simulink model "sistema"  (R2023a)
settings: Solver=ode23t  StartTime=0.0  StopTime=10.0  MaxStep=1e-3  RelTol=1e-6
libraries: fl_lib x18, nesl_utility x9, ee_lib x3, slpidlib x2
settings Model: Creator=Bricia Arellano  LastModifiedBy=Bricia Arellano
settings DataIOCC: ReturnWorkspaceOutputs=off  TimeSaveName=t
settings DebuggingCC: AlgebraicLoopMsg=none  ArtificialAlgebraicLoopMsg=none  MaxConsecutiveZCsMsg=none  ModelReferenceExtraNoncontSigs=none  OperatingPointInterfaceChecksumMismatchMsg=none

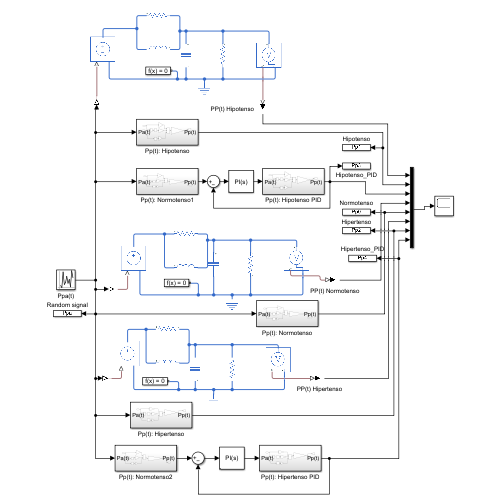
[thumbnail: Simulink's stored preview of the top-level diagram]
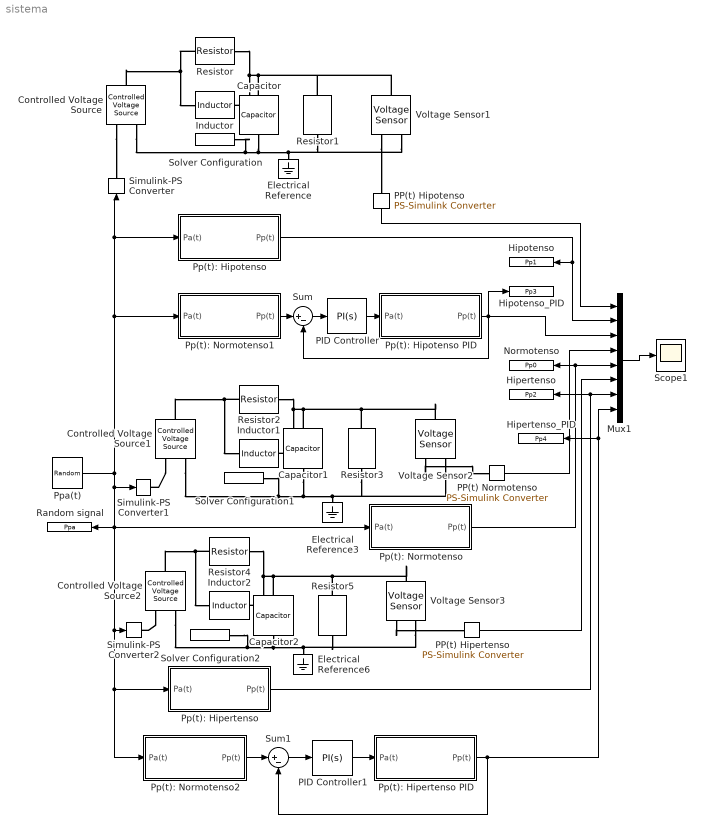
== system sistema ==
  Capacitor : fl_lib/Electrical/Electrical Elements/Capacitor  c=0.25 F  r=1e-6 Ohm  g=0 1/Ohm  i_specify=off  i_priority=None  i=0 A  i_nominal_specify=off  i_nominal_unit=A  i_nominal_value=1  v_specify=off  v_priority=None  v=0 V  v_nominal_specify=off  v_nominal_unit=V  v_nominal_value=1  vc_specify=off  vc_priority=High  vc=0 V  vc_nominal_specify=off  vc_nominal_unit=V  vc_nominal_value=1
  Capacitor1 : fl_lib/Electrical/Electrical Elements/Capacitor  c=1.5 F  r=1e-6 Ohm  g=0 1/Ohm  i_specify=off  i_priority=None  i=0 A  i_nominal_specify=off  i_nominal_unit=A  i_nominal_value=1  v_specify=off  v_priority=None  v=0 V  v_nominal_specify=off  v_nominal_unit=V  v_nominal_value=1  vc_specify=off  vc_priority=High  vc=0 V  vc_nominal_specify=off  vc_nominal_unit=V  vc_nominal_value=1
  Capacitor2 : fl_lib/Electrical/Electrical Elements/Capacitor  c=2.5 F  r=1e-6 Ohm  g=0 1/Ohm  i_specify=off  i_priority=None  i=0 A  i_nominal_specify=off  i_nominal_unit=A  i_nominal_value=1  v_specify=off  v_priority=None  v=0 V  v_nominal_specify=off  v_nominal_unit=V  v_nominal_value=1  vc_specify=off  vc_priority=High  vc=0 V  vc_nominal_specify=off  vc_nominal_unit=V  vc_nominal_value=1
  Controlled Voltage Source : fl_lib/Electrical/Electrical Sources/Controlled Voltage Source
  Controlled Voltage Source1 : fl_lib/Electrical/Electrical Sources/Controlled Voltage Source
  Controlled Voltage Source2 : fl_lib/Electrical/Electrical Sources/Controlled Voltage Source
  Electrical Reference : fl_lib/Electrical/Electrical Elements/Electrical Reference
  Electrical Reference3 : fl_lib/Electrical/Electrical Elements/Electrical Reference
  Electrical Reference6 : fl_lib/Electrical/Electrical Elements/Electrical Reference
  Hipertenso : ToWorkspace  VariableName=Pp2  SampleTime=-1
  Hipertenso_PID : ToWorkspace  VariableName=Pp4  SampleTime=-1
  Hipotenso : ToWorkspace  VariableName=Pp1  SampleTime=-1
  Hipotenso_PID : ToWorkspace  VariableName=Pp3  SampleTime=-1
  Inductor : ee_lib/Passive/Inductor  l=0.005 H  enable_L_tol=ee.enum.toleranceApplication.none  L_tol=20  tol_distribution=ee.enum.toleranceDistribution.uniform  nSigma=4  r=0 Ohm  g=1e-9 1/Ohm  enable_operating_limits=ee.enum.enable.no  operating_limit_action=ee.enum.passive.reportOpLim.warn  max_working_current=1 A  power_rating=1 W  enable_faults=ee.enum.enable.no  fault_action=simscape.enum.assert.action.none  lambdaPercent=50  k_faulted=0.9999  turnsShort=ee.enum.passive.inductor.turnsShortOption.no  openCct=ee.enum.enable.no  groundShort=ee.enum.passive.inductor.groundShortOption.no  groundShortG=0 1/Ohm  tau_fault=1e-3 s  fault_trigger=ee.enum.faults.faultTrigger.temporal  t_fault=1 s  max_permissible_voltage=100 V  n_fail_on_voltage=1  max_permissible_current=1 A  t_fail_on_current=1 s  i_L_specify=off  i_L_priority=High  i_L=0 A  i_L_nominal_specify=off  i_L_nominal_unit=A  i_L_nominal_value=1
  Inductor1 : ee_lib/Passive/Inductor  l=0.01 H  enable_L_tol=ee.enum.toleranceApplication.none  L_tol=20  tol_distribution=ee.enum.toleranceDistribution.uniform  nSigma=4  r=0 Ohm  g=1e-9 1/Ohm  enable_operating_limits=ee.enum.enable.no  operating_limit_action=ee.enum.passive.reportOpLim.warn  max_working_current=1 A  power_rating=1 W  enable_faults=ee.enum.enable.no  fault_action=simscape.enum.assert.action.none  lambdaPercent=50  k_faulted=0.9999  turnsShort=ee.enum.passive.inductor.turnsShortOption.no  openCct=ee.enum.enable.no  groundShort=ee.enum.passive.inductor.groundShortOption.no  groundShortG=0 1/Ohm  tau_fault=1e-3 s  fault_trigger=ee.enum.faults.faultTrigger.temporal  t_fault=1 s  max_permissible_voltage=100 V  n_fail_on_voltage=1  max_permissible_current=1 A  t_fail_on_current=1 s  i_L_specify=off  i_L_priority=High  i_L=0 A  i_L_nominal_specify=off  i_L_nominal_unit=A  i_L_nominal_value=1
  Inductor2 : ee_lib/Passive/Inductor  l=0.02 H  enable_L_tol=ee.enum.toleranceApplication.none  L_tol=20  tol_distribution=ee.enum.toleranceDistribution.uniform  nSigma=4  r=0 Ohm  g=1e-9 1/Ohm  enable_operating_limits=ee.enum.enable.no  operating_limit_action=ee.enum.passive.reportOpLim.warn  max_working_current=1 A  power_rating=1 W  enable_faults=ee.enum.enable.no  fault_action=simscape.enum.assert.action.none  lambdaPercent=50  k_faulted=0.9999  turnsShort=ee.enum.passive.inductor.turnsShortOption.no  openCct=ee.enum.enable.no  groundShort=ee.enum.passive.inductor.groundShortOption.no  groundShortG=0 1/Ohm  tau_fault=1e-3 s  fault_trigger=ee.enum.faults.faultTrigger.temporal  t_fault=1 s  max_permissible_voltage=100 V  n_fail_on_voltage=1  max_permissible_current=1 A  t_fail_on_current=1 s  i_L_specify=off  i_L_priority=High  i_L=0 A  i_L_nominal_specify=off  i_L_nominal_unit=A  i_L_nominal_value=1
  Mux1 : Mux  Inputs=8
  Normotenso : ToWorkspace  VariableName=Pp0  SampleTime=-1
  PID Controller : slpidlib/PID Controller  Controller=PI  Form=Parallel  TimeDomain=Continuous-time  UseExternalTs=off  SampleTime=-1  IntegratorMethod=Forward Euler  FilterMethod=Forward Euler  ControllerParametersSource=internal  P=4.21636346738391e-05  I=3267.68674685278  UseKiTs=off  D=0  N=100  UseFilter=on  TunerSelectOption=Transfer Function Based (PID Tuner App)  InitialConditionSource=internal  InitialConditionForIntegrator=0  InitialConditionForFilter=0  DifferentiatorICPrevScaledInput=0  ExternalReset=none  TrackingMode=off  Kt=1  LimitOutput=off  SatLimitsSource=internal  UpperSaturationLimit=inf  LowerSaturationLimit=-inf  LinearizeAsGain=on  AntiWindupMode=none  Kb=1  LimitIntegrator=off  UpperIntegratorSaturationLimit=inf  LowerIntegratorSaturationLimit=-inf  POutMin=[]  POutMax=[]  IOutMin=[]  IOutMax=[]  DOutMin=[]  DOutMax=[]  NOutMin=[]  NOutMax=[]  SumOutMin=[]  SumOutMax=[]  SaturationOutMin=[]  SaturationOutMax=[]  PParamMin=[]  PParamMax=[]  IParamMin=[]  IParamMax=[]  DParamMin=[]  DParamMax=[]  NParamMin=[]  NParamMax=[]  KbParamMin=[]  KbParamMax=[]  KtParamMin=[]  KtParamMax=[]  KbOutMin=[]  KbOutMax=[]  KtOutMin=[]  KtOutMax=[]  IntegratorOutMin=[]  IntegratorOutMax=[]  FilterOutMin=[]  FilterOutMax=[]  SumI1OutMin=[]  SumI1OutMax=[]  SumI2OutMin=[]  SumI2OutMax=[]  SumI3OutMin=[]  SumI3OutMax=[]  SumI4OutMin=[]  SumI4OutMax=[]  SumDOutMin=[]  SumDOutMax=[]  DifferentiatorOutMin=[]  DifferentiatorOutMax=[]  FilterDiffOutCoefMin=[]  FilterDiffOutCoefMax=[]  ReciprocalOutMin=[]  ReciprocalOutMax=[]  SumDenOutMin=[]  SumDenOutMax=[]  SumNumOutMin=[]  SumNumOutMax=[]  DivideOutMin=[]  DivideOutMax=[]  UdiffTsProdOutMin=[]  UdiffTsProdOutMax=[]  NTsProdOutMin=[]  NTsProdOutMax=[]  UintegralTsProdOutMin=[]  UintegralTsProdOutMax=[]  UngainTsProdOutMin=[]  UngainTsProdOutMax=[]  ClampingZeroOutDataTypeStr=Inherit: Inherit via back propagation  ClampingZeroOutMin=[]  ClampingZeroOutMax=[]  FilterDenConstantOutDataTypeStr=Inherit: Inherit via back propagation  FilterDenConstantOutMin=[]  FilterDenConstantOutMax=[]  PCopyOutDataTypeStr=Inherit: Inherit via back propagation  PCopyOutMin=[]  PCopyOutMax=[]  NCopyOutDataTypeStr=Inherit: Inherit via back propagation  NCopyOutMin=[]  NCopyOutMax=[]  IntegratorContinuousStateAttributes=''  IntegratorStateMustResolveToSignalObject=off  IntegratorRTWStateStorageClass=Auto  FilterContinuousStateAttributes=''  FilterStateMustResolveToSignalObject=off  FilterRTWStateStorageClass=Auto  ParallelPVariant=InternalParameters  IdealPVariant=Disabled  IVariant=InternalParameters  DVariant=Disabled  IntegratorVariant=Continuous  SatVariant=Disabled  AWVariant=Passthrough  PCopyVariant=Disabled  TRVariant=Disabled  FdbkBlocksVariant=Forward  IdealPFdbkVariant=Disabled  SatFdbkVariant=Disabled  DerivativeFilterVariant=Disabled  NVariant=Disabled  NCopyVariant=Disabled_SignalSpec  FilterICVariant=Disabled  IntegratorICVariant=InternalICs  ExternalResetVariant=Disabled  TRSumVariant=Passthrough  SumFdbkVariant=Disabled  SumVariant=Sum_PI  TsampFilterVariant=InternalTs  TsampNgainVariant=Passthrough  TsampIntegralVariant=Disabled_SignalSpec  ExternalSaturationOutDataTypeStr=Inherit: Same as second input
  PID Controller1 : slpidlib/PID Controller  Controller=PI  Form=Parallel  TimeDomain=Continuous-time  UseExternalTs=off  SampleTime=-1  IntegratorMethod=Forward Euler  FilterMethod=Forward Euler  ControllerParametersSource=internal  P=10  I=3275.21614803153  UseKiTs=off  D=0  N=100  UseFilter=on  TunerSelectOption=Transfer Function Based (PID Tuner App)  InitialConditionSource=internal  InitialConditionForIntegrator=0  InitialConditionForFilter=0  DifferentiatorICPrevScaledInput=0  ExternalReset=none  TrackingMode=off  Kt=1  LimitOutput=off  SatLimitsSource=internal  UpperSaturationLimit=inf  LowerSaturationLimit=-inf  LinearizeAsGain=on  AntiWindupMode=none  Kb=1  LimitIntegrator=off  UpperIntegratorSaturationLimit=inf  LowerIntegratorSaturationLimit=-inf  POutMin=[]  POutMax=[]  IOutMin=[]  IOutMax=[]  DOutMin=[]  DOutMax=[]  NOutMin=[]  NOutMax=[]  SumOutMin=[]  SumOutMax=[]  SaturationOutMin=[]  SaturationOutMax=[]  PParamMin=[]  PParamMax=[]  IParamMin=[]  IParamMax=[]  DParamMin=[]  DParamMax=[]  NParamMin=[]  NParamMax=[]  KbParamMin=[]  KbParamMax=[]  KtParamMin=[]  KtParamMax=[]  KbOutMin=[]  KbOutMax=[]  KtOutMin=[]  KtOutMax=[]  IntegratorOutMin=[]  IntegratorOutMax=[]  FilterOutMin=[]  FilterOutMax=[]  SumI1OutMin=[]  SumI1OutMax=[]  SumI2OutMin=[]  SumI2OutMax=[]  SumI3OutMin=[]  SumI3OutMax=[]  SumI4OutMin=[]  SumI4OutMax=[]  SumDOutMin=[]  SumDOutMax=[]  DifferentiatorOutMin=[]  DifferentiatorOutMax=[]  FilterDiffOutCoefMin=[]  FilterDiffOutCoefMax=[]  ReciprocalOutMin=[]  ReciprocalOutMax=[]  SumDenOutMin=[]  SumDenOutMax=[]  SumNumOutMin=[]  SumNumOutMax=[]  DivideOutMin=[]  DivideOutMax=[]  UdiffTsProdOutMin=[]  UdiffTsProdOutMax=[]  NTsProdOutMin=[]  NTsProdOutMax=[]  UintegralTsProdOutMin=[]  UintegralTsProdOutMax=[]  UngainTsProdOutMin=[]  UngainTsProdOutMax=[]  ClampingZeroOutDataTypeStr=Inherit: Inherit via back propagation  ClampingZeroOutMin=[]  ClampingZeroOutMax=[]  FilterDenConstantOutDataTypeStr=Inherit: Inherit via back propagation  FilterDenConstantOutMin=[]  FilterDenConstantOutMax=[]  PCopyOutDataTypeStr=Inherit: Inherit via back propagation  PCopyOutMin=[]  PCopyOutMax=[]  NCopyOutDataTypeStr=Inherit: Inherit via back propagation  NCopyOutMin=[]  NCopyOutMax=[]  IntegratorContinuousStateAttributes=''  IntegratorStateMustResolveToSignalObject=off  IntegratorRTWStateStorageClass=Auto  FilterContinuousStateAttributes=''  FilterStateMustResolveToSignalObject=off  FilterRTWStateStorageClass=Auto  ParallelPVariant=InternalParameters  IdealPVariant=Disabled  IVariant=InternalParameters  DVariant=Disabled  IntegratorVariant=Continuous  SatVariant=Disabled  AWVariant=Passthrough  PCopyVariant=Disabled  TRVariant=Disabled  FdbkBlocksVariant=Forward  IdealPFdbkVariant=Disabled  SatFdbkVariant=Disabled  DerivativeFilterVariant=Disabled  NVariant=Disabled  NCopyVariant=Disabled_SignalSpec  FilterICVariant=Disabled  IntegratorICVariant=InternalICs  ExternalResetVariant=Disabled  TRSumVariant=Passthrough  SumFdbkVariant=Disabled  SumVariant=Sum_PI  TsampFilterVariant=InternalTs  TsampNgainVariant=Passthrough  TsampIntegralVariant=Disabled_SignalSpec  ExternalSaturationOutDataTypeStr=Inherit: Same as second input
  PP(t) Hipertenso : nesl_utility/PS-Simulink Converter  PhysicalDomain=network_engine_domain  SubClassName=ps_output  LeftPortType=input  RightPortType=output  PseudoPeriodic=off  Frequencies=[]  VectorFormat=inherit  Unit=inherit  AffineConversion=off
  PP(t) Hipotenso : nesl_utility/PS-Simulink Converter  PhysicalDomain=network_engine_domain  SubClassName=ps_output  LeftPortType=input  RightPortType=output  PseudoPeriodic=off  Frequencies=[]  VectorFormat=inherit  Unit=inherit  AffineConversion=off
  PP(t) Normotenso : nesl_utility/PS-Simulink Converter  PhysicalDomain=network_engine_domain  SubClassName=ps_output  LeftPortType=input  RightPortType=output  PseudoPeriodic=off  Frequencies=[]  VectorFormat=inherit  Unit=inherit  AffineConversion=off
  Pp(t): Hipertenso : Subsystem
  Pp(t): Hipertenso PID : Subsystem
  Pp(t): Hipotenso : Subsystem
  Pp(t): Hipotenso PID : Subsystem
  Pp(t): Normotenso : Subsystem
  Pp(t): Normotenso1 : Subsystem
  Pp(t): Normotenso2 : Subsystem
  Ppa(t) : UniformRandomNumber  Minimum=-0.2  Seed=106  SampleTime=0.5
  Random signal : ToWorkspace  VariableName=Ppa  SampleTime=-1
  Resistor : fl_lib/Electrical/Electrical Elements/Resistor  R=0.02 Ohm  i_specify=off  i_priority=None  i=0 A  i_nominal_specify=off  i_nominal_unit=A  i_nominal_value=1  v_specify=off  v_priority=None  v=0 V  v_nominal_specify=off  v_nominal_unit=V  v_nominal_value=1
  Resistor1 : fl_lib/Electrical/Electrical Elements/Resistor  R=0.6 Ohm  i_specify=off  i_priority=None  i=0 A  i_nominal_specify=off  i_nominal_unit=A  i_nominal_value=1  v_specify=off  v_priority=None  v=0 V  v_nominal_specify=off  v_nominal_unit=V  v_nominal_value=1
  Resistor2 : fl_lib/Electrical/Electrical Elements/Resistor  R=0.033 Ohm  i_specify=off  i_priority=None  i=0 A  i_nominal_specify=off  i_nominal_unit=A  i_nominal_value=1  v_specify=off  v_priority=None  v=0 V  v_nominal_specify=off  v_nominal_unit=V  v_nominal_value=1
  Resistor3 : fl_lib/Electrical/Electrical Elements/Resistor  R=0.95 Ohm  i_specify=off  i_priority=None  i=0 A  i_nominal_specify=off  i_nominal_unit=A  i_nominal_value=1  v_specify=off  v_priority=None  v=0 V  v_nominal_specify=off  v_nominal_unit=V  v_nominal_value=1
  Resistor4 : fl_lib/Electrical/Electrical Elements/Resistor  R=0.05 Ohm  i_specify=off  i_priority=None  i=0 A  i_nominal_specify=off  i_nominal_unit=A  i_nominal_value=1  v_specify=off  v_priority=None  v=0 V  v_nominal_specify=off  v_nominal_unit=V  v_nominal_value=1
  Resistor5 : fl_lib/Electrical/Electrical Elements/Resistor  R=1.4 Ohm  i_specify=off  i_priority=None  i=0 A  i_nominal_specify=off  i_nominal_unit=A  i_nominal_value=1  v_specify=off  v_priority=None  v=0 V  v_nominal_specify=off  v_nominal_unit=V  v_nominal_value=1
  Scope1 : Scope
  Simulink-PS Converter : nesl_utility/Simulink-PS Converter  PhysicalDomain=network_engine_domain  SubClassName=ps_input  LeftPortType=input  RightPortType=output  PseudoPeriodic=off  Frequencies=[]  NoiseDistribution=none  NoiseParameters=[]  Unit=1  AffineConversion=off  FilteringAndDerivatives=provide  SimscapeFilterOrder=1  InputFilterTimeConstant=0.001  UdotUserProvided=0
  Simulink-PS Converter1 : nesl_utility/Simulink-PS Converter  PhysicalDomain=network_engine_domain  SubClassName=ps_input  LeftPortType=input  RightPortType=output  PseudoPeriodic=off  Frequencies=[]  NoiseDistribution=none  NoiseParameters=[]  Unit=1  AffineConversion=off  FilteringAndDerivatives=provide  SimscapeFilterOrder=1  InputFilterTimeConstant=0.001  UdotUserProvided=0
  Simulink-PS Converter2 : nesl_utility/Simulink-PS Converter  PhysicalDomain=network_engine_domain  SubClassName=ps_input  LeftPortType=input  RightPortType=output  PseudoPeriodic=off  Frequencies=[]  NoiseDistribution=none  NoiseParameters=[]  Unit=1  AffineConversion=off  FilteringAndDerivatives=provide  SimscapeFilterOrder=1  InputFilterTimeConstant=0.001  UdotUserProvided=0
  Solver Configuration : nesl_utility/Solver Configuration  PhysicalDomain=network_engine_domain  SubClassName=solver  LeftPortType=input  RightPortType=generic  Tones=[]  Harmonics=[]  SimulateNoise=off  Profile=off  UseLocalSampling=off  EnableSwitchedLinearOptims=on  FrequencyDomain=off  UseCCode=off  RelTol=0.001  AbsTol=0.001  MinStep=1e-09  ToWorkspace=off  RevertToSquareIcSolve=off  NumHomotopyIterations=100  PhasorMode=off  PhasorModeNumHarmonics=1  ConsistencySolver=NEWTON_XTOL_AFTER_FTOL  IndexReductionMethod=DerivativeReplacement  DoDC=off  ResidualTolerance=1e-09  ConsistencyTolSource=GLOBAL  ConsistencyAbsTol=0.001  ConsistencyRelTol=0.001  ConsistencyTolFactor=0.001  UseLocalSolver=off  LocalSolverChoice=NE_BACKWARD_EULER_ADVANCER  ResolveIndetEquations=on  FunctionEvalNumThread=1  LocalSolverSampleTime=0.001  DoFixedCost=off  MaxNonlinIter=3  MaxModeIter=2  ComputeImpulses=off  ImpulseIterations=2  LinearAlgebra=auto  LinearAlgebraNumThread=0  EquationFormulation=NE_TIME_EF  DelaysMemoryBudget=1024  AutomaticFiltering=on  FilteringTimeConstant=0.001  PartitionStorageMethod=AS_NEEDED  PartitionMemoryBudget=1024  PartitionMethod=ROBUST
  Solver Configuration1 : nesl_utility/Solver Configuration  PhysicalDomain=network_engine_domain  SubClassName=solver  LeftPortType=input  RightPortType=generic  Tones=[]  Harmonics=[]  SimulateNoise=off  Profile=off  UseLocalSampling=off  EnableSwitchedLinearOptims=on  FrequencyDomain=off  UseCCode=off  RelTol=0.001  AbsTol=0.001  MinStep=1e-09  ToWorkspace=off  RevertToSquareIcSolve=off  NumHomotopyIterations=100  PhasorMode=off  PhasorModeNumHarmonics=1  ConsistencySolver=NEWTON_XTOL_AFTER_FTOL  IndexReductionMethod=DerivativeReplacement  DoDC=off  ResidualTolerance=1e-09  ConsistencyTolSource=GLOBAL  ConsistencyAbsTol=0.001  ConsistencyRelTol=0.001  ConsistencyTolFactor=0.001  UseLocalSolver=off  LocalSolverChoice=NE_BACKWARD_EULER_ADVANCER  ResolveIndetEquations=on  FunctionEvalNumThread=1  LocalSolverSampleTime=0.001  DoFixedCost=off  MaxNonlinIter=3  MaxModeIter=2  ComputeImpulses=off  ImpulseIterations=2  LinearAlgebra=auto  LinearAlgebraNumThread=0  EquationFormulation=NE_TIME_EF  DelaysMemoryBudget=1024  AutomaticFiltering=on  FilteringTimeConstant=0.001  PartitionStorageMethod=AS_NEEDED  PartitionMemoryBudget=1024  PartitionMethod=ROBUST
  Solver Configuration2 : nesl_utility/Solver Configuration  PhysicalDomain=network_engine_domain  SubClassName=solver  LeftPortType=input  RightPortType=generic  Tones=[]  Harmonics=[]  SimulateNoise=off  Profile=off  UseLocalSampling=off  EnableSwitchedLinearOptims=on  FrequencyDomain=off  UseCCode=off  RelTol=0.001  AbsTol=0.001  MinStep=1e-09  ToWorkspace=off  RevertToSquareIcSolve=off  NumHomotopyIterations=100  PhasorMode=off  PhasorModeNumHarmonics=1  ConsistencySolver=NEWTON_XTOL_AFTER_FTOL  IndexReductionMethod=DerivativeReplacement  DoDC=off  ResidualTolerance=1e-09  ConsistencyTolSource=GLOBAL  ConsistencyAbsTol=0.001  ConsistencyRelTol=0.001  ConsistencyTolFactor=0.001  UseLocalSolver=off  LocalSolverChoice=NE_BACKWARD_EULER_ADVANCER  ResolveIndetEquations=on  FunctionEvalNumThread=1  LocalSolverSampleTime=0.001  DoFixedCost=off  MaxNonlinIter=3  MaxModeIter=2  ComputeImpulses=off  ImpulseIterations=2  LinearAlgebra=auto  LinearAlgebraNumThread=0  EquationFormulation=NE_TIME_EF  DelaysMemoryBudget=1024  AutomaticFiltering=on  FilteringTimeConstant=0.001  PartitionStorageMethod=AS_NEEDED  PartitionMemoryBudget=1024  PartitionMethod=ROBUST
  Sum : Sum  Inputs=|+-
  Sum1 : Sum  Inputs=|+-
  Voltage Sensor1 : fl_lib/Electrical/Electrical Sensors/Voltage Sensor
  Voltage Sensor2 : fl_lib/Electrical/Electrical Sensors/Voltage Sensor
  Voltage Sensor3 : fl_lib/Electrical/Electrical Sensors/Voltage Sensor
  wires:
  Mux1/1 -> Scope1/1
  Ppa(t)/1 -> Simulink-PS Converter1/1, Random signal/1, Simulink-PS Converter2/1, Pp(t): Hipertenso/1(Pa(t)), Pp(t): Normotenso2/1(Pa(t)), Pp(t): Normotenso/1(Pa(t)), Pp(t): Normotenso1/1(Pa(t)), Pp(t): Hipotenso/1(Pa(t)), Simulink-PS Converter/1
  Pp(t): Hipertenso/1(Pp(t)) -> Hipertenso/1, Mux1/7
  Pp(t): Normotenso/1(Pp(t)) -> Normotenso/1, Mux1/5
  Pp(t): Hipotenso/1(Pp(t)) -> Hipotenso/1, Mux1/2
  PP(t) Hipotenso/1 -> Mux1/1
  PP(t) Normotenso/1 -> Mux1/4
  PP(t) Hipertenso/1 -> Mux1/6
  PID Controller/1 -> Pp(t): Hipotenso PID/1(Pa(t))
  Sum/1 -> PID Controller/1
  Pp(t): Normotenso1/1(Pp(t)) -> Sum/1
  Pp(t): Hipotenso PID/1(Pp(t)) -> Sum/2, Hipotenso_PID/1, Mux1/3
  Sum1/1 -> PID Controller1/1
  PID Controller1/1 -> Pp(t): Hipertenso PID/1(Pa(t))
  Pp(t): Normotenso2/1(Pp(t)) -> Sum1/1
  Pp(t): Hipertenso PID/1(Pp(t)) -> Sum1/2, Mux1/8, Hipertenso_PID/1
  connections:
  Resistor/RConn1 -- Resistor1/LConn1 -- Voltage Sensor1/LConn1 -- Capacitor/LConn1 -- Inductor/RConn1
  Resistor/LConn1 -- Controlled Voltage Source/LConn1 -- Inductor/LConn1
  Voltage Sensor1/RConn1 -- PP(t) Hipotenso/LConn1
  Controlled Voltage Source/RConn1 -- Simulink-PS Converter/RConn1
  Resistor2/LConn1 -- Inductor1/LConn1 -- Controlled Voltage Source1/LConn1
  Resistor3/LConn1 -- Voltage Sensor2/LConn1 -- Capacitor1/LConn1 -- Inductor1/RConn1 -- Resistor2/RConn1
  Controlled Voltage Source1/RConn1 -- Simulink-PS Converter1/RConn1
  Resistor5/LConn1 -- Voltage Sensor3/LConn1 -- Capacitor2/LConn1 -- Inductor2/RConn1 -- Resistor4/RConn1
  Resistor4/LConn1 -- Controlled Voltage Source2/LConn1 -- Inductor2/LConn1
  Controlled Voltage Source2/RConn1 -- Simulink-PS Converter2/RConn1
  Voltage Sensor3/RConn1 -- PP(t) Hipertenso/LConn1
  Voltage Sensor2/RConn1 -- PP(t) Normotenso/LConn1
  Controlled Voltage Source/RConn2 -- Solver Configuration/RConn1 -- Capacitor/RConn1 -- Resistor1/RConn1 -- Voltage Sensor1/RConn2 -- Electrical Reference/LConn1
  Controlled Voltage Source1/RConn2 -- Solver Configuration1/RConn1 -- Capacitor1/RConn1 -- Resistor3/RConn1 -- Voltage Sensor2/RConn2 -- Electrical Reference3/LConn1
  Controlled Voltage Source2/RConn2 -- Solver Configuration2/RConn1 -- Capacitor2/RConn1 -- Resistor5/RConn1 -- Voltage Sensor3/RConn2 -- Electrical Reference6/LConn1

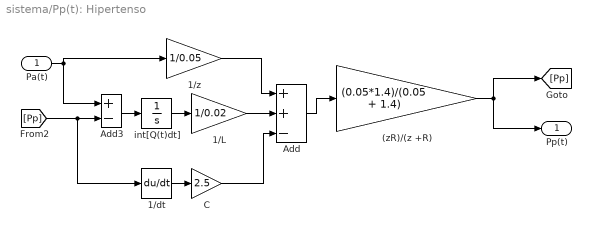
== system sistema/Pp(t): Hipertenso ==
  Pa(t) : Inport
  (zR)/(z +R) : Gain  Gain=(0.05*1.4)/(0.05 + 1.4)
  1/L : Gain  Gain=1/0.02
  1/dt : Derivative
  1/z : Gain  Gain=1/0.05
  Add : Sum  Inputs=++-
  Add3 : Sum  Inputs=+-
  C : Gain  Gain=2.5
  int[Q(t)dt] : Integrator
  Pp(t) : Outport
  wires:
  Add/1 -> (zR)/(z +R)/1
  (zR)/(z +R)/1 -> [Pp], Pp(t)/1
  [Pp] -> 1/dt/1, Add3/2
  1/L/1 -> Add/2
  Pa(t)/1 -> Add3/1, 1/z/1
  1/z/1 -> Add/1
  1/dt/1 -> C/1
  C/1 -> Add/3
  int[Q(t)dt]/1 -> 1/L/1
  Add3/1 -> int[Q(t)dt]/1

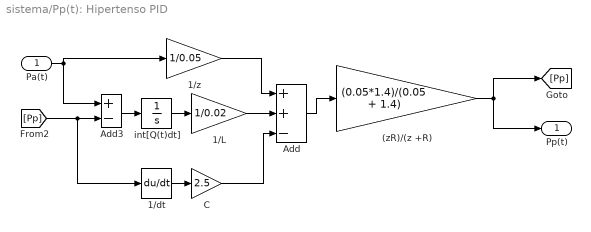
== system sistema/Pp(t): Hipertenso PID ==
  Pa(t) : Inport
  (zR)/(z +R) : Gain  Gain=(0.05*1.4)/(0.05 + 1.4)
  1/L : Gain  Gain=1/0.02
  1/dt : Derivative
  1/z : Gain  Gain=1/0.05
  Add : Sum  Inputs=++-
  Add3 : Sum  Inputs=+-
  C : Gain  Gain=2.5
  int[Q(t)dt] : Integrator
  Pp(t) : Outport
  wires:
  Add/1 -> (zR)/(z +R)/1
  (zR)/(z +R)/1 -> [Pp], Pp(t)/1
  [Pp] -> 1/dt/1, Add3/2
  1/L/1 -> Add/2
  Pa(t)/1 -> Add3/1, 1/z/1
  1/z/1 -> Add/1
  1/dt/1 -> C/1
  C/1 -> Add/3
  int[Q(t)dt]/1 -> 1/L/1
  Add3/1 -> int[Q(t)dt]/1

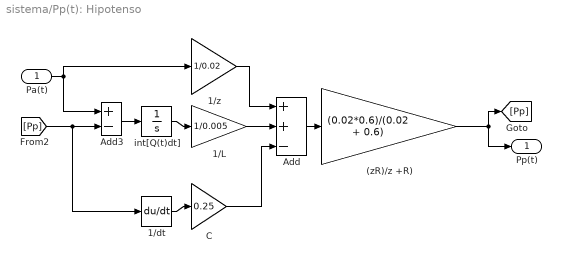
== system sistema/Pp(t): Hipotenso ==
  Pa(t) : Inport
  (zR)/z +R) : Gain  Gain=(0.02*0.6)/(0.02 + 0.6)
  1/L : Gain  Gain=1/0.005
  1/dt : Derivative
  1/z : Gain  Gain=1/0.02
  Add : Sum  Inputs=++-
  Add3 : Sum  Inputs=+-
  C : Gain  Gain=0.25
  int[Q(t)dt] : Integrator
  Pp(t) : Outport
  wires:
  Add/1 -> (zR)/z +R)/1
  (zR)/z +R)/1 -> Pp(t)/1, [Pp]
  [Pp] -> 1/dt/1, Add3/2
  1/L/1 -> Add/2
  Pa(t)/1 -> Add3/1, 1/z/1
  1/z/1 -> Add/1
  1/dt/1 -> C/1
  C/1 -> Add/3
  int[Q(t)dt]/1 -> 1/L/1
  Add3/1 -> int[Q(t)dt]/1

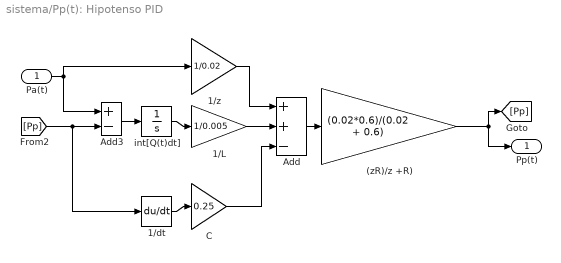
== system sistema/Pp(t): Hipotenso PID ==
  Pa(t) : Inport
  (zR)/z +R) : Gain  Gain=(0.02*0.6)/(0.02 + 0.6)
  1/L : Gain  Gain=1/0.005
  1/dt : Derivative
  1/z : Gain  Gain=1/0.02
  Add : Sum  Inputs=++-
  Add3 : Sum  Inputs=+-
  C : Gain  Gain=0.25
  int[Q(t)dt] : Integrator
  Pp(t) : Outport
  wires:
  Add/1 -> (zR)/z +R)/1
  (zR)/z +R)/1 -> Pp(t)/1, [Pp]
  [Pp] -> 1/dt/1, Add3/2
  1/L/1 -> Add/2
  Pa(t)/1 -> Add3/1, 1/z/1
  1/z/1 -> Add/1
  1/dt/1 -> C/1
  C/1 -> Add/3
  int[Q(t)dt]/1 -> 1/L/1
  Add3/1 -> int[Q(t)dt]/1

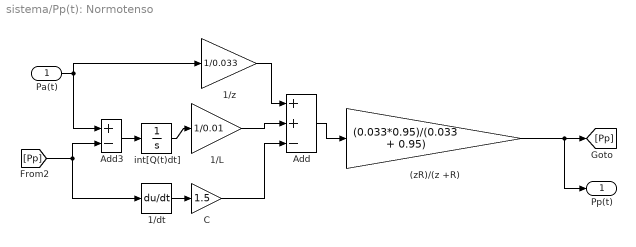
== system sistema/Pp(t): Normotenso ==
  Pa(t) : Inport
  (zR)/(z +R) : Gain  Gain=(0.033*0.95)/(0.033 + 0.95)
  1/L : Gain  Gain=1/0.01
  1/dt : Derivative
  1/z : Gain  Gain=1/0.033
  Add : Sum  Inputs=++-
  Add3 : Sum  Inputs=+-
  C : Gain  Gain=1.5
  int[Q(t)dt] : Integrator
  Pp(t) : Outport
  wires:
  Add/1 -> (zR)/(z +R)/1
  (zR)/(z +R)/1 -> Pp(t)/1, [Pp]
  [Pp] -> 1/dt/1, Add3/2
  1/L/1 -> Add/2
  Pa(t)/1 -> Add3/1, 1/z/1
  1/z/1 -> Add/1
  1/dt/1 -> C/1
  C/1 -> Add/3
  int[Q(t)dt]/1 -> 1/L/1
  Add3/1 -> int[Q(t)dt]/1

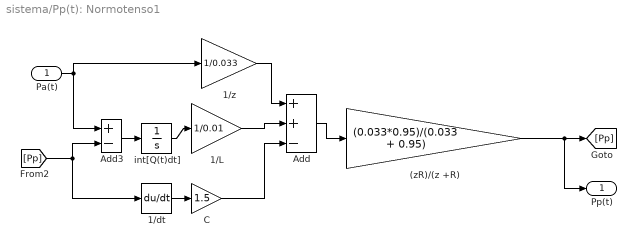
== system sistema/Pp(t): Normotenso1 ==
  Pa(t) : Inport
  (zR)/(z +R) : Gain  Gain=(0.033*0.95)/(0.033 + 0.95)
  1/L : Gain  Gain=1/0.01
  1/dt : Derivative
  1/z : Gain  Gain=1/0.033
  Add : Sum  Inputs=++-
  Add3 : Sum  Inputs=+-
  C : Gain  Gain=1.5
  int[Q(t)dt] : Integrator
  Pp(t) : Outport
  wires:
  Add/1 -> (zR)/(z +R)/1
  (zR)/(z +R)/1 -> Pp(t)/1, [Pp]
  [Pp] -> 1/dt/1, Add3/2
  1/L/1 -> Add/2
  Pa(t)/1 -> Add3/1, 1/z/1
  1/z/1 -> Add/1
  1/dt/1 -> C/1
  C/1 -> Add/3
  int[Q(t)dt]/1 -> 1/L/1
  Add3/1 -> int[Q(t)dt]/1

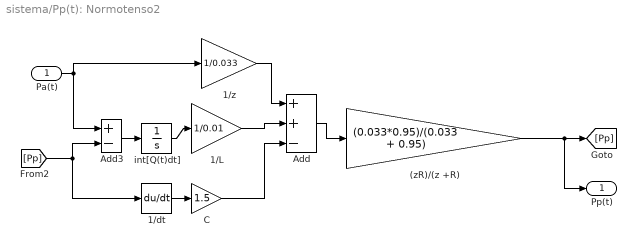
== system sistema/Pp(t): Normotenso2 ==
  Pa(t) : Inport
  (zR)/(z +R) : Gain  Gain=(0.033*0.95)/(0.033 + 0.95)
  1/L : Gain  Gain=1/0.01
  1/dt : Derivative
  1/z : Gain  Gain=1/0.033
  Add : Sum  Inputs=++-
  Add3 : Sum  Inputs=+-
  C : Gain  Gain=1.5
  int[Q(t)dt] : Integrator
  Pp(t) : Outport
  wires:
  Add/1 -> (zR)/(z +R)/1
  (zR)/(z +R)/1 -> Pp(t)/1, [Pp]
  [Pp] -> 1/dt/1, Add3/2
  1/L/1 -> Add/2
  Pa(t)/1 -> Add3/1, 1/z/1
  1/z/1 -> Add/1
  1/dt/1 -> C/1
  C/1 -> Add/3
  int[Q(t)dt]/1 -> 1/L/1
  Add3/1 -> int[Q(t)dt]/1
